simulink model "Variable_Size_Signal"  (R2024a)
settings: Solver=VariableStepAuto  StartTime=0.0  StopTime=20  RelTol=1e-3
libraries: simulink x1, aieUtilities x1
settings Model: Creator=abehbood  LastModifiedBy=robg
settings SolverCC: AlgebraicLoopSolver=TrustRegion
settings DebuggingCC: UnconnectedInputMsg=warning  UnconnectedOutputMsg=warning  UnconnectedLineMsg=warning
settings ModelReferenceCC: EnableRefExpFcnMdlSchedulingChecks=on
settings RTWCC: GPUComputeCapability=3.5
settings ConfigComp: CovBoundaryAbsTol=1.0e-5

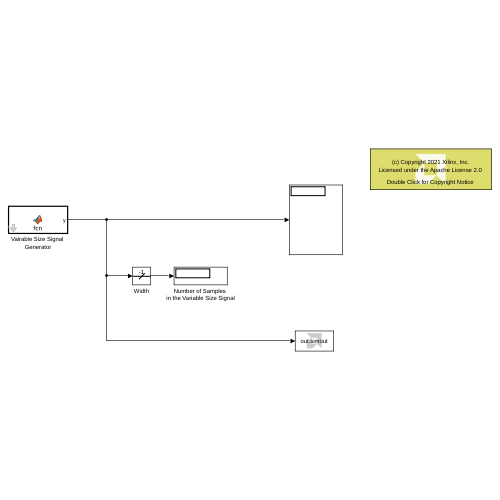
[thumbnail: Simulink's stored preview of the top-level diagram]
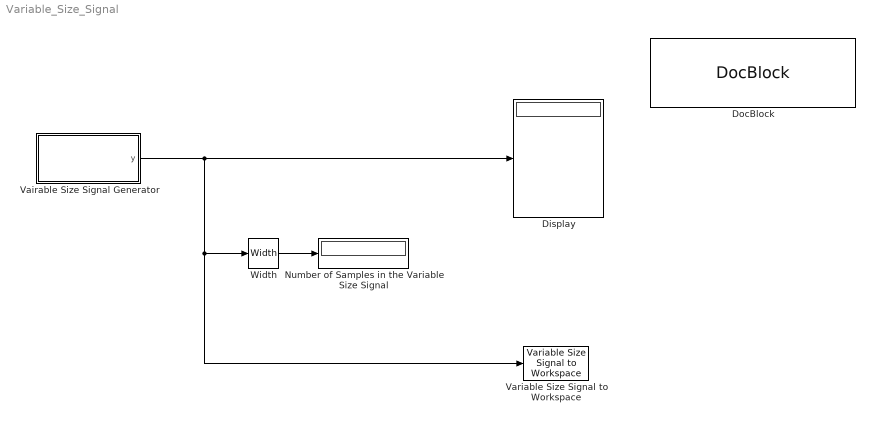
== system Variable_Size_Signal ==
  Display : Display
  DocBlock : simulink/Model-Wide Utilities/DocBlock  DocumentType=Text  mask(DocBlock){}
      content=|
      | ///////////////////////////////////////////////////////////////////////////
      | // Copyright 2021 Xilinx
      | //
      | // Licensed under the Apache License, Version 2.0 (the "License");
      | // you may not use this file except in compliance with the License.
      | // You may obtain a copy of the License at
      | //
      | // http://www.apache.org/licenses/LICENSE-2.0
      | //
      | // Unless required by applicable law or agreed to in writing, software
      | // distributed under the License is distributed on an "AS IS" BASIS,
      | // WITHOUT WARRANTIES OR CONDITIONS OF ANY KIND, either express or implied.
      | // See the License for the specific language governing permissions and
      | // limitations under the License.
      | ///////////////////////////////////////////////////////////////////////////
      mask Display:
      | xmcDrawBlockIcon();
      | disp(['{\fontsize{10pt}(c) Copyright 2021' ' Xilinx, Inc.}\newline \newline '],'texmode','on');
      | disp('{\fontsize{10pt}Licensed under the Apache License 2.0}','texmode','on');
      | disp('\newline \newline \newline{\fontsize{10pt}Double Click for Copyright Notice}','texmode','on');
  Number of Samples in the Variable Size Signal : Display
  Vairable Size Signal Generator : MATLAB Function  TreatAsAtomicUnit=on  SystemSampleTime=1  mask{maxSizeOfVariableSizeSignal=4, outType=Random}
      mask prompts: maxSizeOfVariableSizeSignal "Max Size of Variabel Size Signal"; outType "Number of elements in the output"
      mask help: This block generates a variable size signal output. The number of samples in the output can be random or fixed and are consecutive integer numbers starting from zero.
  Variable Size Signal to Workspace : aieUtilities/Variable Size Signal to Workspace  VariableNameMask=simout
  Width : Width
  wires:
  Vairable Size Signal Generator/1(y) -> Variable Size Signal to Workspace/1, Width/1, Display/1
  Width/1 -> Number of Samples in the Variable Size Signal/1

== matlab function Variable_Size_Signal/Vairable Size Signal Generator ==
  data: y output size=maxSizeOfVariableSizeSignal; maxSizeOfVariableSizeSignal parameter; outType parameter
function y = fcn(maxSizeOfVariableSizeSignal,outType)
%#codegen

persistent out;

if isempty(out)
    out = 0;
    rng(5)
end

if outType == 1
    numOfSamples = randi([0 maxSizeOfVariableSizeSignal],1,1);
else
    numOfSamples = maxSizeOfVariableSizeSignal;
end

y = (out:out+numOfSamples-1)';

out = out + numOfSamples;
